simulink model "interface"  (R2018b)
settings: Solver=FixedStepDiscrete  StartTime=0.0  StopTime=10.0  RelTol=1e-3
settings Model: Creator=matlab  LastModifiedBy=matlab

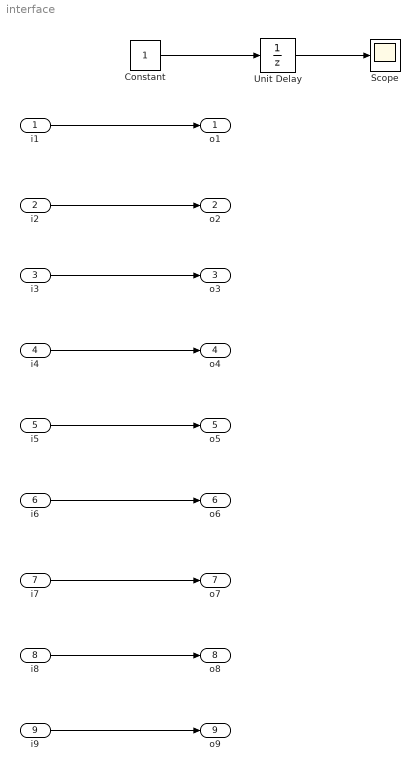
== system interface ==
  i1 : Inport  OutDataTypeStr=AliasToAliasDouble  PortDimensions=[2 2]
  i2 : Inport  Port=2  OutDataTypeStr=AliasToAliasSingle  PortDimensions=[2 2]
  i3 : Inport  Port=3  OutDataTypeStr=AliasToAliasInt8  PortDimensions=[2 2]
  i4 : Inport  Port=4  OutDataTypeStr=AliasToAliasUInt8  PortDimensions=[2 2]
  i5 : Inport  Port=5  OutDataTypeStr=AliasToAliasInt16  PortDimensions=[2 2]
  i6 : Inport  Port=6  OutDataTypeStr=AliasToAliasUInt16  PortDimensions=[2 2]
  i7 : Inport  Port=7  OutDataTypeStr=AliasToAliasInt32  PortDimensions=[2 2]
  i8 : Inport  Port=8  OutDataTypeStr=AliasToAliasUInt32  PortDimensions=[2 2]
  i9 : Inport  Port=9  OutDataTypeStr=AliasToAliasBoolean  PortDimensions=[2 2]
  Constant : Constant
  Scope : Scope
  Unit Delay : UnitDelay  SampleTime=-1
  o1 : Outport  OutDataTypeStr=AliasToAliasDouble  PortDimensions=[2 2]
  o2 : Outport  Port=2  OutDataTypeStr=AliasToAliasSingle  PortDimensions=[2 2]
  o3 : Outport  Port=3  OutDataTypeStr=AliasToAliasInt8  PortDimensions=[2 2]
  o4 : Outport  Port=4  OutDataTypeStr=AliasToAliasUInt8  PortDimensions=[2 2]
  o5 : Outport  Port=5  OutDataTypeStr=AliasToAliasInt16  PortDimensions=[2 2]
  o6 : Outport  Port=6  OutDataTypeStr=AliasToAliasUInt16  PortDimensions=[2 2]
  o7 : Outport  Port=7  OutDataTypeStr=AliasToAliasInt32  PortDimensions=[2 2]
  o8 : Outport  Port=8  OutDataTypeStr=AliasToAliasUInt32  PortDimensions=[2 2]
  o9 : Outport  Port=9  OutDataTypeStr=AliasToAliasBoolean  PortDimensions=[2 2]
  wires:
  i2/1 -> o2/1
  i3/1 -> o3/1
  i4/1 -> o4/1
  i5/1 -> o5/1
  i6/1 -> o6/1
  i7/1 -> o7/1
  i8/1 -> o8/1
  i9/1 -> o9/1
  i1/1 -> o1/1
  Unit Delay/1 -> Scope/1
  Constant/1 -> Unit Delay/1
